simulink model "B2B_2x15kW_LCO_paralelo_y_serie"  (R2026b)
settings: Solver=ode5  StopTime=inf  EnableMultiTasking=on
StopFcn:
  | Modelo_Disable_B2B
undefined symbols (not defined in the file): ALPHA_DC, COS_RO, dataStateMachine, DiscIntNeverNeededParam, dq2abc, EN_G, getNormalizedOffset, I_MAX_G, INV_SIN_RO, KAW_CCG, KAW_DC, KI_CCG, KI_DC, KI_PLLG, KP_CCG, KP_DC, KP_PLLG, L12, LIMIT_SAG_DETECT, magnitude, MIN_VDC_READY, Ncount, NDELAY_SAG_DETECT, PORC_DC_STEADS, SAMPLES_SAG_DETECT, simDCcontCurrent1, simDCcontCurrent2, SN_G, Transformations_blocks, ts, Ts_al, TS_C, TS_PLL, UDC_min_al, UDC_Ref_al, VDC_REF, WN_G
libraries: simulink x15, TriPhaseDriveControl x13, powerlib_extras x2, model_hardware_PM15F80C_rev x2, TriphaseXenomaiTarget x1
(part 1 of 4)
settings Model: ExtModeArchiveDirName=C:\Users\erick.vazquez\Desktop\Modelos serie-paralelo LCOs-FLL  ExtModeArchiveFileName=Inicializacion_paralelo_serie  ExtModeTrigDirection=either  ExtModeTrigElement=1  SimulationMode=external  Creator=francisco.huerta  LastModifiedBy=ERICK
settings DataIOCC: LimitDataPoints=on  ReturnWorkspaceOutputs=off  SaveFormat=Array  SignalLoggingSaveFormat=ModelDataLogs
settings OptimizationCC: BlockReduction=off  BufferReuse=off  ExpressionFolding=off  GlobalBufferReuse=off  LifeSpan=inf  LocalBlockOutputs=off  OptimizeBlockIOStorage=off
settings DebuggingCC: ArithmeticOperatorsInVariantConditions=warning  MergeDetectMultiDrivingBlocksExec=none  MultiTaskCondExecSysMsg=none  MultiTaskDSMMsg=warning  SFExecutionAtInitializationDiag=none  SFNoUnconditionalDefaultTransitionDiag=warning  SFUnexpectedBacktrackingDiag=warning  SolverPrmCheckMsg=warning  StateNameClashWarn=warning  UnderspecifiedInitializationDetection=Classic
settings HardwareCC: ProdEndianess=Unspecified  ProdHWDeviceType=Generic->64-bit Embedded Processor (LP64)  ProdIntDivRoundTo=Undefined  ProdLargestAtomicFloat=None
settings ModelReferenceCC: PropagateSignalLabelsOutOfModel=off
settings SFSimCC: CustomCodeUndefinedFunction=UseInterfaceOnly  SimUseLocalCustomCode=off
settings RTWCC: Description=Linux/Xenomai Native Real-Time Target  RTWUseLocalCustomCode=off  SystemTargetFile=xenomai.tlc  TemplateMakefile=xenomai.tmf
settings CodeAppCC: StateflowObjectComments=on
settings STFCustomTargetCC: CPPClassGenCompliant=on  CodeReplacementLibrary=GNU  ModelReferenceCompliant=off  SystemTargetFile=xenomai.tlc
settings GRTTargetCC: CodeReplacementLibrary=GNU  CombineOutputUpdateFcns=off  CompOptLevelCompliant=off  ConcurrentExecutionCompliant=off  ExtMode=on  ExtModeMexArgs='10.0.14.31', 0, 17725  GRTInterface=on  MatFileLogging=off  ModelReferenceCompliant=off  ParMdlRefBuildCompliant=off
settings ConfigComp: CovExternalEMLEnable=off  CovSFcnEnable=off  CovSaveCumulativeToWorkspaceVar=on  CovSaveSingleToWorkspaceVar=on

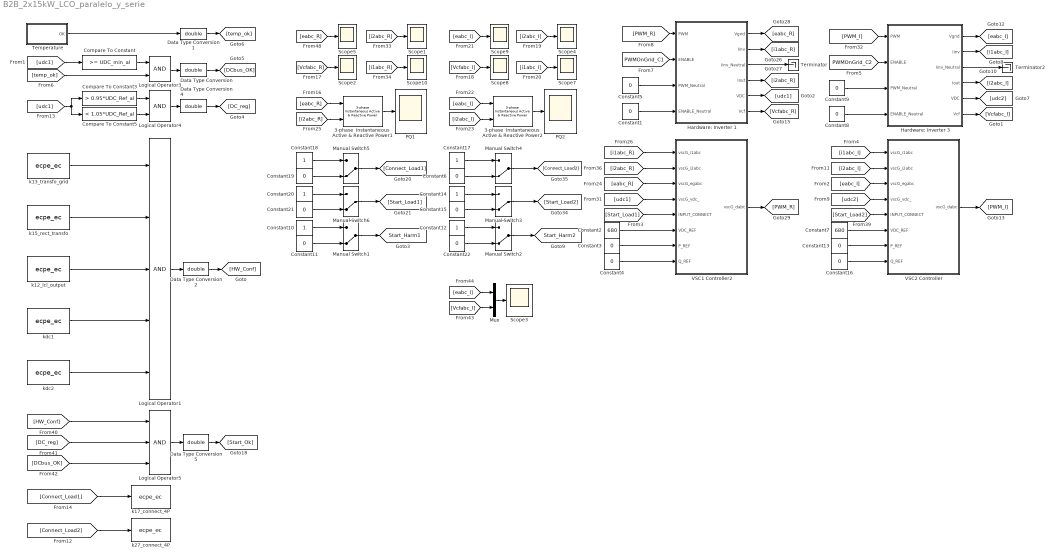
== system B2B_2x15kW_LCO_paralelo_y_serie ==
  3-phase  Instantaneous  Active & Reactive Power1 : powerlib_extras/Measurements/3-phase  Instantaneous  Active & Reactive Power
  3-phase  Instantaneous  Active & Reactive Power2 : powerlib_extras/Measurements/3-phase  Instantaneous  Active & Reactive Power
  Compare To Constant : simulink/Logic and Bit Operations/Compare To Constant  relop=>=  const=UDC_min_al  OutDataTypeStr=boolean
  Compare To Constant3 : simulink/Logic and Bit Operations/Compare To Constant  relop=>  const=0.95*UDC_Ref_al  OutDataTypeStr=boolean
  Compare To Constant5 : simulink/Logic and Bit Operations/Compare To Constant  relop=<  const=1.05*UDC_Ref_al  OutDataTypeStr=boolean
  Constant{1,3..6,8..9,11,13,15..16,19,21..22} (14 alike) : Constant  Value=0
  Constant{10,12,14,17..18,20} (6 alike) : Constant
  Constant2 : Constant  Value=680
  Constant7 : Constant  Value=680
  Data Type Conversion{,1..2,4..5} (5 alike) : DataTypeConversion  OutDataTypeStr=double  SaturateOnIntegerOverflow=off  RndMeth=Floor
  Hardware: Inverter 1 : Subsystem
  Hardware: Inverter 3 : Subsystem
  Logical Operator1 : Logic  Inputs=5  AllPortsSameDT=off  OutDataTypeStr=boolean  SampleTime=Ts_al
  Logical Operator3 : Logic  AllPortsSameDT=off  OutDataTypeStr=boolean  SampleTime=Ts_al
  Logical Operator4 : Logic  AllPortsSameDT=off  OutDataTypeStr=boolean  SampleTime=Ts_al
  Logical Operator5 : Logic  Inputs=3  AllPortsSameDT=off  OutDataTypeStr=boolean  SampleTime=Ts_al
  Manual Switch{1..6} (6 alike) : ManualSwitch  CurrentSetting=0
  Mux : Mux  Inputs=2
  PQ1 : Scope
      settings: TimeSpan=1  ActiveDisplayYMinimum=-200  ActiveDisplayYMaximum=1200  DataLoggingMaxPoints=10000  DataLoggingVariableName=Potencias_C1
  PQ2 : Scope
      settings: TimeSpan=10  ActiveDisplayYMinimum=-1750  ActiveDisplayYMaximum=3000  DataLoggingMaxPoints=10000  DataLoggingVariableName=Potencias_C2
  Scope{1..5,7..10} (9 alike) : Scope
      Scope1 settings: TimeSpan=0.1  ActiveDisplayYMinimum=-6  ActiveDisplayYMaximum=6  DataLoggingVariableName=I2_1_abc
      Scope10 settings: TimeSpan=0.1  DataLoggingVariableName=MedidasTrifasicas1
      Scope2 settings: TimeSpan=0.04  ActiveDisplayYMinimum=-400  ActiveDisplayYMaximum=400  DataLoggingVariableName=MedidasTrifasicas3
      Scope3 settings: TimeSpan=0.04  ActiveDisplayYMinimum=-700  ActiveDisplayYMaximum=800  DataLoggingVariableName=MedidasTrifasicas
      Scope4 settings: TimeSpan=0.04  ActiveDisplayYMinimum=-3.5  ActiveDisplayYMaximum=4  DataLoggingVariableName=I2_2_abc
      Scope5 settings: TimeSpan=0.04  ActiveDisplayYMinimum=-350  ActiveDisplayYMaximum=350  DataLoggingVariableName=Vpcc1_abc
      Scope7 settings: TimeSpan=0.1  ActiveDisplayYMinimum=-0.45  ActiveDisplayYMaximum=0.025  DataLoggingVariableName=MedidasTrifasicas5
      Scope8 settings: TimeSpan=0.1  ActiveDisplayYMinimum=-0.5  ActiveDisplayYMaximum=3.5  DataLoggingVariableName=MedidasTrifasicas6
      Scope9 settings: TimeSpan=0.04  ActiveDisplayYMinimum=-2  ActiveDisplayYMaximum=6  DataLoggingVariableName=Vpcc2_abc
  Temperature : Subsystem
  Terminator : Terminator
  Terminator2 : Terminator
  VSC1 Controller2 : Subsystem
  VSC2 Controller : Subsystem
  k12_lcl_output : TriPhaseDriveControl/Hardware/ecpe_ec  sampletime=Ts_al  names_out='k12_lcl_output'  names_in=''  use_default_values=on  out_values=[]
  k13_transfo_grid : TriPhaseDriveControl/Hardware/ecpe_ec  sampletime=Ts_al  names_out='k13_transfo_grid'  names_in=''  use_default_values=on  out_values=[]
  k15_rect_transfo : TriPhaseDriveControl/Hardware/ecpe_ec  sampletime=Ts_al  names_out='k15_rect_transfo'  names_in=''  use_default_values=on  out_values=[]
  k17_connect_4P : TriPhaseDriveControl/Hardware/ecpe_ec  sampletime=Ts_al  names_out=''  names_in='k17_connect_4P'  use_default_values=on  out_values=[]
  k27_connect_4P : TriPhaseDriveControl/Hardware/ecpe_ec  sampletime=Ts_al  names_out=''  names_in='k27_connect_4P'  use_default_values=on  out_values=[]
  kdc1 : TriPhaseDriveControl/Hardware/ecpe_ec  sampletime=Ts_al  names_out='kdc1'  names_in=''  use_default_values=on  out_values=[]
  kdc2 : TriPhaseDriveControl/Hardware/ecpe_ec  sampletime=Ts_al  names_out='kdc2'  names_in=''  use_default_values=on  out_values=[]
  tag scope: Start_Harm1=global, Start_Harm2=global
  wires:
  Logical Operator1/1 -> Data Type Conversion2/1
  [udc1] -> Compare To Constant/1
  Compare To Constant/1 -> Logical Operator3/1
  Logical Operator3/1 -> Data Type Conversion/1
  [temp_ok] -> Logical Operator3/2
  Temperature/1(OK) -> Data Type Conversion1/1
  Data Type Conversion/1 -> [DCbus_OK]
  Data Type Conversion1/1 -> [temp_ok]
  Data Type Conversion2/1 -> [HW_Conf]
  [udc1] -> Compare To Constant3/1, Compare To Constant5/1
  Compare To Constant3/1 -> Logical Operator4/1
  Compare To Constant5/1 -> Logical Operator4/2
  Data Type Conversion4/1 -> [DC_reg]
  Logical Operator4/1 -> Data Type Conversion4/1
  [Vcfabc_R] -> Scope2/1
  [eabc_R] -> Scope5/1
  Constant5/1 -> Hardware: Inverter 1/3(PWM_Neutral)
  Constant1/1 -> Hardware: Inverter 1/4(ENABLE_Neutral)
  Hardware: Inverter 1/1(Vgrid) -> [eabc_R]
  Hardware: Inverter 1/2(Iinv) -> [i1abc_R]
  Hardware: Inverter 1/3(Iinv_Neutral) -> Terminator/1
  Hardware: Inverter 1/4(Iout) -> [i2abc_R]
  Hardware: Inverter 1/5(VDC) -> [udc1]
  Hardware: Inverter 1/6(Vcf) -> [Vcfabc_R]
  Manual Switch3/1 -> [Start_Load2]
  Manual Switch4/1 -> [Connect_Load2]
  Constant14/1 -> Manual Switch3/1
  Constant15/1 -> Manual Switch3/2
  Constant6/1 -> Manual Switch4/2
  Constant17/1 -> Manual Switch4/1
  [i2abc_R] -> Scope1/1
  Hardware: Inverter 3/1(Vgrid) -> [eabc_I]
  Hardware: Inverter 3/4(Iout) -> [i2abc_I]
  Hardware: Inverter 3/2(Iinv) -> [i1abc_I]
  Hardware: Inverter 3/6(Vcf) -> [Vcfabc_I]
  Hardware: Inverter 3/5(VDC) -> [udc2]
  Hardware: Inverter 3/3(Iinv_Neutral) -> Terminator2/1
  Constant9/1 -> Hardware: Inverter 3/3(PWM_Neutral)
  Constant8/1 -> Hardware: Inverter 3/4(ENABLE_Neutral)
  [eabc_R] -> 3-phase  Instantaneous  Active & Reactive Power1/1
  [i2abc_R] -> 3-phase  Instantaneous  Active & Reactive Power1/2
  3-phase  Instantaneous  Active & Reactive Power1/1 -> PQ1/1
  [i1abc_R] -> Scope10/1
  VSC2 Controller/1(vscG_dabc) -> [PWM_I]
  [i1abc_I] -> VSC2 Controller/1(vscG_i1abc)
  [i2abc_I] -> VSC2 Controller/2(vscG_i2abc)
  [eabc_I] -> VSC2 Controller/3(vscG_egabc)
  [udc2] -> VSC2 Controller/4(vscG_vdc_)
  Constant16/1 -> VSC2 Controller/8(Q_REF)
  Constant13/1 -> VSC2 Controller/7(P_REF)
  [Connect_Load2] -> k27_connect_4P/1
  [Vcfabc_I] -> Scope8/1
  [eabc_I] -> Scope9/1
  [i2abc_I] -> Scope4/1
  [i1abc_I] -> Scope7/1
  [eabc_I] -> 3-phase  Instantaneous  Active & Reactive Power2/1
  [i2abc_I] -> 3-phase  Instantaneous  Active & Reactive Power2/2
  3-phase  Instantaneous  Active & Reactive Power2/1 -> PQ2/1
  [Start_Load2] -> VSC2 Controller/5(INPUT_CONNECT)
  [HW_Conf] -> Logical Operator5/1
  [DC_reg] -> Logical Operator5/2
  [DCbus_OK] -> Logical Operator5/3
  Logical Operator5/1 -> Data Type Conversion5/1
  Data Type Conversion5/1 -> [Start_Ok]
  Manual Switch5/1 -> [Connect_Load1]
  Manual Switch6/1 -> [Start_Load1]
  Constant18/1 -> Manual Switch5/1
  Constant19/1 -> Manual Switch5/2
  Constant21/1 -> Manual Switch6/2
  Constant20/1 -> Manual Switch6/1
  Mux/1 -> Scope3/1
  [eabc_I] -> Mux/1
  [Vcfabc_I] -> Mux/2
  [Connect_Load1] -> k17_connect_4P/1
  VSC1 Controller2/1(vscG_dabc) -> [PWM_R]
  Constant3/1 -> VSC1 Controller2/7(P_REF)
  Constant4/1 -> VSC1 Controller2/8(Q_REF)
  [i2abc_R] -> VSC1 Controller2/2(vscG_i2abc)
  [Start_Load1] -> VSC1 Controller2/5(INPUT_CONNECT)
  [i1abc_R] -> VSC1 Controller2/1(vscG_i1abc)
  [udc1] -> VSC1 Controller2/4(vscG_vdc_)
  [eabc_R] -> VSC1 Controller2/3(vscG_egabc)
  Constant2/1 -> VSC1 Controller2/6(VDC_REF)
  Constant7/1 -> VSC2 Controller/6(VDC_REF)
  k13_transfo_grid/1 -> Logical Operator1/1
  k15_rect_transfo/1 -> Logical Operator1/2
  k12_lcl_output/1 -> Logical Operator1/3
  kdc2/1 -> Logical Operator1/5
  kdc1/1 -> Logical Operator1/4
  [PWMOnGrid_C1] -> Hardware: Inverter 1/2(ENABLE)
  [PWMOnGrid_C2] -> Hardware: Inverter 3/2(ENABLE)
  [PWM_R] -> Hardware: Inverter 1/1(PWM)
  [PWM_I] -> Hardware: Inverter 3/1(PWM)
  Manual Switch1/1 -> [Start_Harm1]
  Constant11/1 -> Manual Switch1/2
  Constant10/1 -> Manual Switch1/1
  Manual Switch2/1 -> [Start_Harm2]
  Constant22/1 -> Manual Switch2/2
  Constant12/1 -> Manual Switch2/1

== system B2B_2x15kW_LCO_paralelo_y_serie/Hardware: Inverter 1 ==
  PWM : Inport
  ENABLE : Inport  Port=2
  PWM_Neutral : Inport  Port=3
  ENABLE_Neutral : Inport  Port=4
  Hardware: 3ph + N (Inverter 1) no termination inv3 : model_hardware_PM15F80C_rev/Hardware: 3ph + N (Inverter 1) no termination inv3  Ts=Ts_al  DT=DT_al  ack=0
  Off-set : Subsystem
  Off-set1 : Subsystem
  Off-set2 : Subsystem
  Off-set3 : Subsystem
  Voltage1 : TriPhaseDriveControl/Hardware/Voltage  Ts=ts  devNames='INVERTER_1/U/M4/CH10,INVERTER_1/U/M4/CH11,INVERTER_1/U/M4/CH12'  vLimOn=off  vLim=600  vFilt=none  vRange=1000  vOffs=getNormalizedOffset([0 0 0], 1000, 1/8000)
  Vgrid : Outport
  Iinv : Outport  Port=2
  Iinv_Neutral : Outport  Port=3
  Iout : Outport  Port=4
  VDC : Outport  Port=5
  Vcf : Outport  Port=6
  wires:
  PWM_Neutral/1 -> Hardware: 3ph + N (Inverter 1) no termination inv3/3
  Hardware: 3ph + N (Inverter 1) no termination inv3/5 -> VDC/1
  ENABLE/1 -> Hardware: 3ph + N (Inverter 1) no termination inv3/2
  PWM/1 -> Hardware: 3ph + N (Inverter 1) no termination inv3/1
  ENABLE_Neutral/1 -> Hardware: 3ph + N (Inverter 1) no termination inv3/4
  Hardware: 3ph + N (Inverter 1) no termination inv3/2 -> Off-set1/1(In)
  Hardware: 3ph + N (Inverter 1) no termination inv3/4 -> Off-set/1(In)
  Hardware: 3ph + N (Inverter 1) no termination inv3/1 -> Off-set2/1(In)
  Voltage1/1 -> Off-set3/1(In)
  Off-set2/1(Out) -> Vgrid/1
  Off-set1/1(Out) -> Iinv/1
  Hardware: 3ph + N (Inverter 1) no termination inv3/3 -> Iinv_Neutral/1
  Off-set/1(Out) -> Iout/1
  Off-set3/1(Out) -> Vcf/1

== system B2B_2x15kW_LCO_paralelo_y_serie/Hardware: Inverter 3 ==
  PWM : Inport
  ENABLE : Inport  Port=2
  PWM_Neutral : Inport  Port=3
  ENABLE_Neutral : Inport  Port=4
  Hardware: 3ph + N (Inverter 3) no termination inv1 : model_hardware_PM15F80C_rev/Hardware: 3ph + N (Inverter 3) no termination inv1  Ts=Ts_al  DT=DT_al  ack=0
  Off-set : Subsystem
  Off-set1 : Subsystem
  Off-set2 : Subsystem
  Off-set3 : Subsystem
  Voltage1 : TriPhaseDriveControl/Hardware/Voltage  Ts=ts  devNames='INVERTER_3/U/M4/CH10,INVERTER_3/U/M4/CH11,INVERTER_3/U/M4/CH12'  vLimOn=off  vLim=600  vFilt=none  vRange=1000  vOffs=getNormalizedOffset([0 0 0], 1000, 1/8000)
  Vgrid : Outport
  Iinv : Outport  Port=2
  Iinv_Neutral : Outport  Port=3
  Iout : Outport  Port=4
  VDC : Outport  Port=5
  Vcf : Outport  Port=6
  wires:
  Voltage1/1 -> Off-set3/1(In)
  Hardware: 3ph + N (Inverter 3) no termination inv1/1 -> Off-set2/1(In)
  Hardware: 3ph + N (Inverter 3) no termination inv1/3 -> Iinv_Neutral/1
  Hardware: 3ph + N (Inverter 3) no termination inv1/4 -> Off-set/1(In)
  Hardware: 3ph + N (Inverter 3) no termination inv1/2 -> Off-set1/1(In)
  ENABLE_Neutral/1 -> Hardware: 3ph + N (Inverter 3) no termination inv1/4
  PWM/1 -> Hardware: 3ph + N (Inverter 3) no termination inv1/1
  ENABLE/1 -> Hardware: 3ph + N (Inverter 3) no termination inv1/2
  Hardware: 3ph + N (Inverter 3) no termination inv1/5 -> VDC/1
  PWM_Neutral/1 -> Hardware: 3ph + N (Inverter 3) no termination inv1/3
  Off-set1/1(Out) -> Iinv/1
  Off-set/1(Out) -> Iout/1
  Off-set2/1(Out) -> Vgrid/1
  Off-set3/1(Out) -> Vcf/1

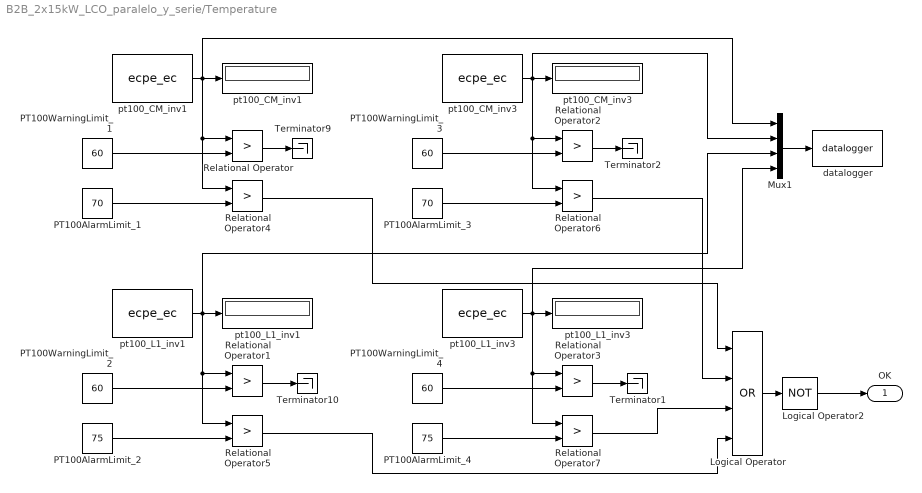
== system B2B_2x15kW_LCO_paralelo_y_serie/Temperature ==
  Logical Operator : Logic  Operator=OR  Inputs=4  AllPortsSameDT=off  OutDataTypeStr=boolean
  Logical Operator2 : Logic  Operator=NOT  AllPortsSameDT=off  OutDataTypeStr=boolean
  Mux1 : Mux
  PT100AlarmLimit_1 : Constant  Value=70
  PT100AlarmLimit_2 : Constant  Value=75
  PT100AlarmLimit_3 : Constant  Value=70
  PT100AlarmLimit_4 : Constant  Value=75
  PT100WarningLimit_{1..4} (4 alike) : Constant  Value=60
  Relational Operator{,1..7} (8 alike) : RelationalOperator  Operator=>  OutDataTypeStr=boolean  InputSameDT=off
  Terminator{1..2,9..10} (4 alike) : Terminator
  datalogger : TriphaseXenomaiTarget/datalogger  memoryName=triphase_temperature  decimation=1/Ts_al*0.5  sampleTime=Ts_al
  pt100_CM_inv1 : TriPhaseDriveControl/Hardware/ecpe_ec  sampletime=Ts_al  names_out='pt100_CM_inv1'  names_in=''  use_default_values=on  out_values=[]
  "pt100_CM_inv1 " : Display
      settings: Decimation=round(0.5/ts)
  pt100_CM_inv3 : TriPhaseDriveControl/Hardware/ecpe_ec  sampletime=Ts_al  names_out='pt100_CM_inv3'  names_in=''  use_default_values=on  out_values=[]
  "pt100_CM_inv3 " : Display
      settings: Decimation=round(0.5/ts)
  pt100_L1_inv1 : TriPhaseDriveControl/Hardware/ecpe_ec  sampletime=Ts_al  names_out='pt100_L1_inv1'  names_in=''  use_default_values=on  out_values=[]
  "pt100_L1_inv1 " : Display
      settings: Decimation=round(0.5/ts)
  pt100_L1_inv3 : TriPhaseDriveControl/Hardware/ecpe_ec  sampletime=Ts_al  names_out='pt100_L1_inv3'  names_in=''  use_default_values=on  out_values=[]
  "pt100_L1_inv3 " : Display
      settings: Decimation=round(0.5/ts)
  OK : Outport
  wires:
  pt100_CM_inv1/1 -> "pt100_CM_inv1 "/1, Relational Operator/1, Relational Operator4/1, Mux1/1
  pt100_L1_inv1/1 -> "pt100_L1_inv1 "/1, Relational Operator1/1, Relational Operator5/1, Mux1/3
  PT100WarningLimit_1/1 -> Relational Operator/2
  Relational Operator/1 -> Terminator9/1
  PT100WarningLimit_2/1 -> Relational Operator1/2
  Relational Operator1/1 -> Terminator10/1
  PT100AlarmLimit_1/1 -> Relational Operator4/2
  PT100AlarmLimit_2/1 -> Relational Operator5/2
  Logical Operator/1 -> Logical Operator2/1
  Logical Operator2/1 -> OK/1
  pt100_CM_inv3/1 -> "pt100_CM_inv3 "/1, Relational Operator2/1, Relational Operator6/1, Mux1/2
  pt100_L1_inv3/1 -> "pt100_L1_inv3 "/1, Relational Operator3/1, Relational Operator7/1, Mux1/4
  PT100WarningLimit_3/1 -> Relational Operator2/2
  Relational Operator2/1 -> Terminator2/1
  PT100WarningLimit_4/1 -> Relational Operator3/2
  Relational Operator3/1 -> Terminator1/1
  PT100AlarmLimit_3/1 -> Relational Operator6/2
  PT100AlarmLimit_4/1 -> Relational Operator7/2
  Relational Operator4/1 -> Logical Operator/1
  Relational Operator6/1 -> Logical Operator/2
  Relational Operator5/1 -> Logical Operator/4
  Relational Operator7/1 -> Logical Operator/3
  Mux1/1 -> datalogger/1

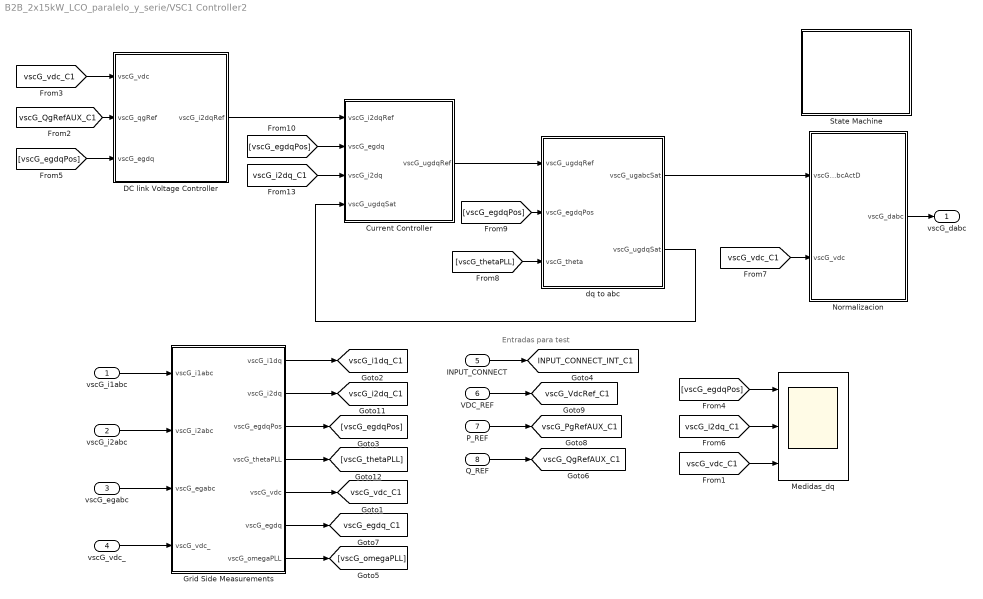
== system B2B_2x15kW_LCO_paralelo_y_serie/VSC1 Controller2 ==
  note: Entradas para test
  vscG_i1abc : Inport  SampleTime=TS_C
  vscG_i2abc : Inport  Port=2  SampleTime=TS_C
  vscG_egabc : Inport  Port=3  SampleTime=TS_PLL
  vscG_vdc_ : Inport  Port=4  SampleTime=TS_C
  INPUT_CONNECT : Inport  Port=5  SampleTime=TS_PLL
  VDC_REF : Inport  Port=6  SampleTime=TS_PLL
  P_REF : Inport  Port=7  SampleTime=TS_PLL
  Q_REF : Inport  Port=8  SampleTime=TS_PLL
  Current Controller : Subsystem
  DC link Voltage Controller : Subsystem
  Grid Side Measurements : Subsystem
  Medidas_dq : Scope  NumInputPorts=3
      settings: TimeSpan=5  ActiveDisplayYMinimum=-200  ActiveDisplayYMaximum=225  DataLoggingVariableName=MedidasDQ_C1
  Normalizacion : Subsystem
  State Machine : Subsystem
  dq to abc : Subsystem
  vscG_dabc : Outport
  tag scope: INPUT_CONNECT_INT_C1=global, vscG_PgRefAUX_C1=global, vscG_QgRefAUX_C1=global, vscG_VdcRef_C1=global, vscG_egdq_C1=global, vscG_i1dq_C1=global, vscG_i2dq_C1=global, vscG_vdc_C1=global
  wires:
  vscG_i1abc/1 -> Grid Side Measurements/1(vscG_i1abc)
  vscG_i2abc/1 -> Grid Side Measurements/2(vscG_i2abc)
  vscG_egabc/1 -> Grid Side Measurements/3(vscG_egabc)
  Grid Side Measurements/3(vscG_egdqPos) -> [vscG_egdqPos]
  DC link Voltage Controller/1(vscG_i2dqRef) -> Current Controller/1(vscG_i2dqRef)
  Current Controller/1(vscG_ugdqRef) -> dq to abc/1(vscG_ugdqRef)
  [vscG_egdqPos] -> DC link Voltage Controller/3(vscG_egdq)
  vscG_vdc_/1 -> Grid Side Measurements/4(vscG_vdc_)
  [vscG_vdc_C1] -> DC link Voltage Controller/1(vscG_vdc)
  Grid Side Measurements/6(vscG_egdq) -> [vscG_egdq_C1]
  Grid Side Measurements/7(vscG_omegaPLL) -> [vscG_omegaPLL]
  Grid Side Measurements/5(vscG_vdc) -> [vscG_vdc_C1]
  [vscG_vdc_C1] -> Normalizacion/2(vscG_vdc)
  Normalizacion/1(vscG_dabc) -> vscG_dabc/1
  INPUT_CONNECT/1 -> [INPUT_CONNECT_INT_C1]
  VDC_REF/1 -> [vscG_VdcRef_C1]
  P_REF/1 -> [vscG_PgRefAUX_C1]
  Q_REF/1 -> [vscG_QgRefAUX_C1]
  Grid Side Measurements/1(vscG_i1dq) -> [vscG_i1dq_C1]
  Grid Side Measurements/4(vscG_thetaPLL) -> [vscG_thetaPLL]
  Grid Side Measurements/2(vscG_i2dq) -> [vscG_i2dq_C1]
  [vscG_egdqPos] -> Current Controller/2(vscG_egdq)
  [vscG_i2dq_C1] -> Current Controller/3(vscG_i2dq)
  [vscG_thetaPLL] -> dq to abc/3(vscG_theta)
  [vscG_QgRefAUX_C1] -> DC link Voltage Controller/2(vscG_qgRef)
  [vscG_vdc_C1] -> Medidas_dq/3
  [vscG_i2dq_C1] -> Medidas_dq/2
  [vscG_egdqPos] -> Medidas_dq/1
  dq to abc/1(vscG_ugabcSat) -> Normalizacion/1(vscG_ugabcActD)
  [vscG_egdqPos] -> dq to abc/2(vscG_egdqPos)
  dq to abc/2(vscG_ugdqSat) -> Current Controller/4(vscG_ugdqSat)

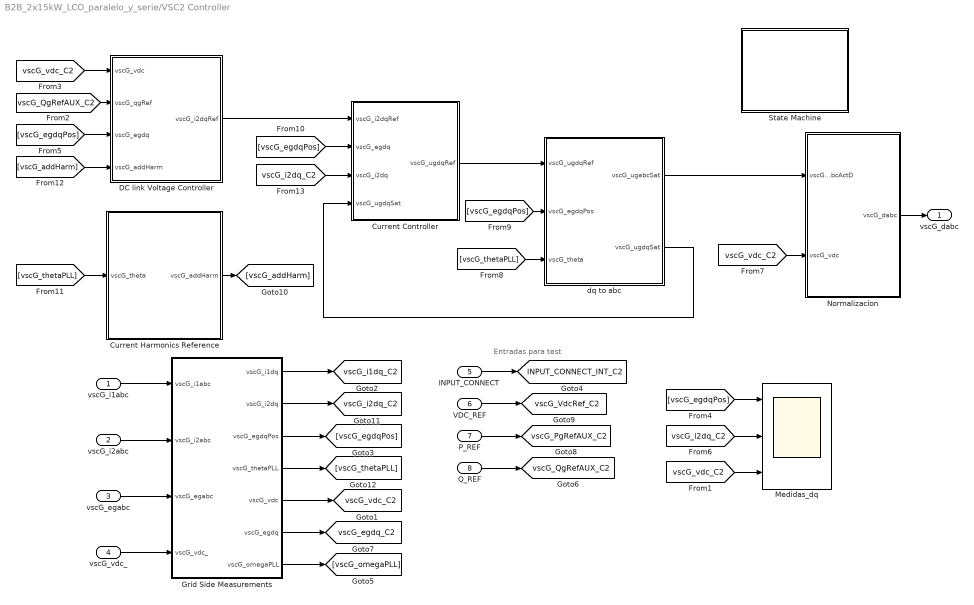
== system B2B_2x15kW_LCO_paralelo_y_serie/VSC2 Controller ==
  note: Entradas para test
  vscG_i1abc : Inport  SampleTime=TS_C
  vscG_i2abc : Inport  Port=2  SampleTime=TS_C
  vscG_egabc : Inport  Port=3  SampleTime=TS_PLL
  vscG_vdc_ : Inport  Port=4  SampleTime=TS_C
  INPUT_CONNECT : Inport  Port=5  SampleTime=TS_PLL
  VDC_REF : Inport  Port=6  SampleTime=TS_PLL
  P_REF : Inport  Port=7  SampleTime=TS_PLL
  Q_REF : Inport  Port=8  SampleTime=TS_PLL
  Current Controller : Subsystem
  Current Harmonics Reference : Subsystem
  DC link Voltage Controller : Subsystem
  Grid Side Measurements : Subsystem
  Medidas_dq : Scope  NumInputPorts=3
      settings: TimeSpan=10  ActiveDisplayYMinimum=320  ActiveDisplayYMaximum=350  DataLoggingVariableName=MedidasDQ_C2
  Normalizacion : Subsystem
  State Machine : Subsystem
  dq to abc : Subsystem
  vscG_dabc : Outport
  tag scope: INPUT_CONNECT_INT_C2=global, vscG_PgRefAUX_C2=global, vscG_QgRefAUX_C2=global, vscG_VdcRef_C2=global, vscG_egdq_C2=global, vscG_i1dq_C2=global, vscG_i2dq_C2=global, vscG_vdc_C2=global
  wires:
  vscG_i1abc/1 -> Grid Side Measurements/1(vscG_i1abc)
  vscG_i2abc/1 -> Grid Side Measurements/2(vscG_i2abc)
  vscG_egabc/1 -> Grid Side Measurements/3(vscG_egabc)
  Grid Side Measurements/3(vscG_egdqPos) -> [vscG_egdqPos]
  DC link Voltage Controller/1(vscG_i2dqRef) -> Current Controller/1(vscG_i2dqRef)
  Current Controller/1(vscG_ugdqRef) -> dq to abc/1(vscG_ugdqRef)
  [vscG_egdqPos] -> DC link Voltage Controller/3(vscG_egdq)
  vscG_vdc_/1 -> Grid Side Measurements/4(vscG_vdc_)
  [vscG_vdc_C2] -> DC link Voltage Controller/1(vscG_vdc)
  Grid Side Measurements/6(vscG_egdq) -> [vscG_egdq_C2]
  Grid Side Measurements/7(vscG_omegaPLL) -> [vscG_omegaPLL]
  Grid Side Measurements/5(vscG_vdc) -> [vscG_vdc_C2]
  [vscG_vdc_C2] -> Normalizacion/2(vscG_vdc)
  Normalizacion/1(vscG_dabc) -> vscG_dabc/1
  INPUT_CONNECT/1 -> [INPUT_CONNECT_INT_C2]
  VDC_REF/1 -> [vscG_VdcRef_C2]
  P_REF/1 -> [vscG_PgRefAUX_C2]
  Q_REF/1 -> [vscG_QgRefAUX_C2]
  Grid Side Measurements/1(vscG_i1dq) -> [vscG_i1dq_C2]
  Grid Side Measurements/4(vscG_thetaPLL) -> [vscG_thetaPLL]
  Grid Side Measurements/2(vscG_i2dq) -> [vscG_i2dq_C2]
  [vscG_egdqPos] -> Current Controller/2(vscG_egdq)
  [vscG_i2dq_C2] -> Current Controller/3(vscG_i2dq)
  [vscG_thetaPLL] -> dq to abc/3(vscG_theta)
  [vscG_QgRefAUX_C2] -> DC link Voltage Controller/2(vscG_qgRef)
  [vscG_vdc_C2] -> Medidas_dq/3
  [vscG_i2dq_C2] -> Medidas_dq/2
  [vscG_egdqPos] -> Medidas_dq/1
  dq to abc/1(vscG_ugabcSat) -> Normalizacion/1(vscG_ugabcActD)
  [vscG_egdqPos] -> dq to abc/2(vscG_egdqPos)
  dq to abc/2(vscG_ugdqSat) -> Current Controller/4(vscG_ugdqSat)
  Current Harmonics Reference/1(vscG_addHarm) -> [vscG_addHarm]
  [vscG_thetaPLL] -> Current Harmonics Reference/1(vscG_theta)
  [vscG_addHarm] -> DC link Voltage Controller/4(vscG_addHarm)

== system B2B_2x15kW_LCO_paralelo_y_serie/Hardware: Inverter 1/Off-set ==
  In : Inport
  Demux1 : Demux  Outputs=3
  Mux1 : Mux  Inputs=3
  Sum : Sum  Inputs=|++
  Sum1 : Sum  Inputs=|++
  Sum2 : Sum  Inputs=|++
  a : Constant  Value=0
  b : Constant  Value=0
  c : Constant  Value=0
  Out : Outport
  wires:
  Mux1/1 -> Out/1
  Demux1/2 -> Sum1/1
  Demux1/1 -> Sum/1
  Sum1/1 -> Mux1/2
  In/1 -> Demux1/1
  Sum/1 -> Mux1/1
  Sum2/1 -> Mux1/3
  Demux1/3 -> Sum2/1
  a/1 -> Sum/2
  b/1 -> Sum1/2
  c/1 -> Sum2/2

== system B2B_2x15kW_LCO_paralelo_y_serie/Hardware: Inverter 1/Off-set1 ==
  In : Inport
  Demux1 : Demux  Outputs=3
  Mux1 : Mux  Inputs=3
  Sum : Sum  Inputs=|++
  Sum1 : Sum  Inputs=|++
  Sum2 : Sum  Inputs=|++
  a : Constant  Value=0
  b : Constant  Value=-0.6
  c : Constant  Value=0.5
  Out : Outport
  wires:
  Mux1/1 -> Out/1
  Demux1/2 -> Sum1/1
  Demux1/1 -> Sum/1
  Sum1/1 -> Mux1/2
  In/1 -> Demux1/1
  Sum/1 -> Mux1/1
  Sum2/1 -> Mux1/3
  Demux1/3 -> Sum2/1
  a/1 -> Sum/2
  b/1 -> Sum1/2
  c/1 -> Sum2/2

== system B2B_2x15kW_LCO_paralelo_y_serie/Hardware: Inverter 1/Off-set2 ==
  In : Inport
  Demux1 : Demux  Outputs=3
  Mux1 : Mux  Inputs=3
  Sum : Sum  Inputs=|++
  Sum1 : Sum  Inputs=|++
  Sum2 : Sum  Inputs=|++
  a : Constant  Value=-3
  b : Constant  Value=-1.5
  c : Constant  Value=0
  Out : Outport
  wires:
  Mux1/1 -> Out/1
  Demux1/2 -> Sum1/1
  Demux1/1 -> Sum/1
  Sum1/1 -> Mux1/2
  In/1 -> Demux1/1
  Sum/1 -> Mux1/1
  Sum2/1 -> Mux1/3
  Demux1/3 -> Sum2/1
  a/1 -> Sum/2
  b/1 -> Sum1/2
  c/1 -> Sum2/2

== system B2B_2x15kW_LCO_paralelo_y_serie/Hardware: Inverter 1/Off-set3 ==
  In : Inport
  Demux1 : Demux  Outputs=3
  Mux1 : Mux  Inputs=3
  Sum : Sum  Inputs=|++
  Sum1 : Sum  Inputs=|++
  Sum2 : Sum  Inputs=|++
  a : Constant  Value=0
  b : Constant  Value=0
  c : Constant  Value=0
  Out : Outport
  wires:
  Mux1/1 -> Out/1
  Demux1/2 -> Sum1/1
  Demux1/1 -> Sum/1
  Sum1/1 -> Mux1/2
  In/1 -> Demux1/1
  Sum/1 -> Mux1/1
  Sum2/1 -> Mux1/3
  Demux1/3 -> Sum2/1
  a/1 -> Sum/2
  b/1 -> Sum1/2
  c/1 -> Sum2/2

== system B2B_2x15kW_LCO_paralelo_y_serie/Hardware: Inverter 3/Off-set ==
  In : Inport
  Demux1 : Demux  Outputs=3
  Mux1 : Mux  Inputs=3
  Sum : Sum  Inputs=|++
  Sum1 : Sum  Inputs=|++
  Sum2 : Sum  Inputs=|++
  a : Constant  Value=0.05
  b : Constant  Value=0.15
  c : Constant  Value=-0.05
  Out : Outport
  wires:
  Mux1/1 -> Out/1
  Demux1/2 -> Sum1/1
  Demux1/1 -> Sum/1
  Sum1/1 -> Mux1/2
  In/1 -> Demux1/1
  Sum/1 -> Mux1/1
  Sum2/1 -> Mux1/3
  Demux1/3 -> Sum2/1
  a/1 -> Sum/2
  b/1 -> Sum1/2
  c/1 -> Sum2/2

== system B2B_2x15kW_LCO_paralelo_y_serie/Hardware: Inverter 3/Off-set1 ==
  In : Inport
  Demux1 : Demux  Outputs=3
  Mux1 : Mux  Inputs=3
  Sum : Sum  Inputs=|++
  Sum1 : Sum  Inputs=|++
  Sum2 : Sum  Inputs=|++
  a : Constant  Value=0.35
  b : Constant  Value=0.05
  c : Constant  Value=0.1
  Out : Outport
  wires:
  Mux1/1 -> Out/1
  Demux1/2 -> Sum1/1
  Demux1/1 -> Sum/1
  Sum1/1 -> Mux1/2
  In/1 -> Demux1/1
  Sum/1 -> Mux1/1
  Sum2/1 -> Mux1/3
  Demux1/3 -> Sum2/1
  a/1 -> Sum/2
  b/1 -> Sum1/2
  c/1 -> Sum2/2

== system B2B_2x15kW_LCO_paralelo_y_serie/Hardware: Inverter 3/Off-set2 ==
  In : Inport
  Demux1 : Demux  Outputs=3
  Mux1 : Mux  Inputs=3
  Sum : Sum  Inputs=|++
  Sum1 : Sum  Inputs=|++
  Sum2 : Sum  Inputs=|++
  a : Constant  Value=3
  b : Constant  Value=0
  c : Constant  Value=2
  Out : Outport
  wires:
  Mux1/1 -> Out/1
  Demux1/2 -> Sum1/1
  Demux1/1 -> Sum/1
  Sum1/1 -> Mux1/2
  In/1 -> Demux1/1
  Sum/1 -> Mux1/1
  Sum2/1 -> Mux1/3
  Demux1/3 -> Sum2/1
  a/1 -> Sum/2
  b/1 -> Sum1/2
  c/1 -> Sum2/2

== system B2B_2x15kW_LCO_paralelo_y_serie/Hardware: Inverter 3/Off-set3 ==
  In : Inport
  Demux1 : Demux  Outputs=3
  Mux1 : Mux  Inputs=3
  Sum : Sum  Inputs=|++
  Sum1 : Sum  Inputs=|++
  Sum2 : Sum  Inputs=|++
  a : Constant
  b : Constant  Value=3.7
  c : Constant  Value=6
  Out : Outport
  wires:
  Mux1/1 -> Out/1
  Demux1/2 -> Sum1/1
  Demux1/1 -> Sum/1
  Sum1/1 -> Mux1/2
  In/1 -> Demux1/1
  Sum/1 -> Mux1/1
  Sum2/1 -> Mux1/3
  Demux1/3 -> Sum2/1
  a/1 -> Sum/2
  b/1 -> Sum1/2
  c/1 -> Sum2/2

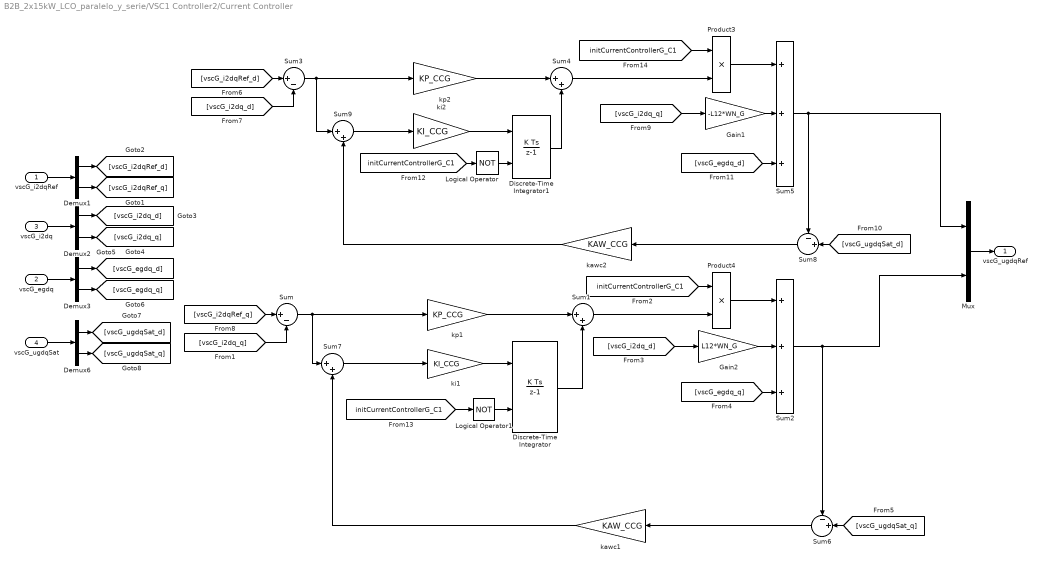
== system B2B_2x15kW_LCO_paralelo_y_serie/VSC1 Controller2/Current Controller ==
  vscG_i2dqRef : Inport
  vscG_egdq : Inport  Port=2
  vscG_i2dq : Inport  Port=3
  vscG_ugdqSat : Inport  Port=4
  Demux{1..3,6} (4 alike) : Demux  Outputs=2
  Discrete-Time Integrator : DiscreteIntegrator  ExternalReset=level  SampleTime=-1  UpperSaturationLimit=sqrt(2/3)*750  LowerSaturationLimit=-sqrt(2/3)*750  ICPrevOutput=DiscIntNeverNeededParam  ICPrevScaledInput=DiscIntNeverNeededParam
  Discrete-Time Integrator1 : DiscreteIntegrator  ExternalReset=level  SampleTime=-1  UpperSaturationLimit=sqrt(2/3)*750  LowerSaturationLimit=-sqrt(2/3)*750  ICPrevOutput=DiscIntNeverNeededParam  ICPrevScaledInput=DiscIntNeverNeededParam
  Gain1 : Gain  Gain=-L12*WN_G  SaturateOnIntegerOverflow=on  OutDataTypeStr=Inherit: Same as input  ParamDataTypeStr=Inherit: Same as input
  Gain2 : Gain  Gain=L12*WN_G  SaturateOnIntegerOverflow=on  OutDataTypeStr=Inherit: Same as input  ParamDataTypeStr=Inherit: Same as input
  Logical Operator : Logic  Operator=NOT  AllPortsSameDT=off  OutDataTypeStr=boolean
  Logical Operator1 : Logic  Operator=NOT  AllPortsSameDT=off  OutDataTypeStr=boolean
  Mux : Mux  Inputs=2
  Product3 : Product  InputSameDT=on  SaturateOnIntegerOverflow=on  OutDataTypeStr=Inherit: Same as first input
  Product4 : Product  InputSameDT=on  SaturateOnIntegerOverflow=on  OutDataTypeStr=Inherit: Same as first input
  Sum : Sum  Inputs=|+-  InputSameDT=on  SaturateOnIntegerOverflow=on  OutDataTypeStr=Inherit: Same as first input
  Sum{1,4,7,9} (4 alike) : Sum  Inputs=|++  InputSameDT=on  SaturateOnIntegerOverflow=on  OutDataTypeStr=Inherit: Same as first input
  Sum2 : Sum  Inputs=+++  InputSameDT=on  SaturateOnIntegerOverflow=on  OutDataTypeStr=Inherit: Same as first input
  Sum3 : Sum  Inputs=|+-  InputSameDT=on  SaturateOnIntegerOverflow=on  OutDataTypeStr=Inherit: Same as first input
  Sum5 : Sum  Inputs=+++  InputSameDT=on  SaturateOnIntegerOverflow=on  OutDataTypeStr=Inherit: Same as first input
  Sum6 : Sum  Inputs=-+|  InputSameDT=on  SaturateOnIntegerOverflow=on  OutDataTypeStr=Inherit: Same as first input
  Sum8 : Sum  Inputs=-+|  InputSameDT=on  SaturateOnIntegerOverflow=on  OutDataTypeStr=Inherit: Same as first input
  kawc1 : Gain  Gain=KAW_CCG  SaturateOnIntegerOverflow=on  OutDataTypeStr=Inherit: Same as input  ParamDataTypeStr=Inherit: Same as input
  kawc2 : Gain  Gain=KAW_CCG  SaturateOnIntegerOverflow=on  OutDataTypeStr=Inherit: Same as input  ParamDataTypeStr=Inherit: Same as input
  ki1 : Gain  Gain=KI_CCG  SaturateOnIntegerOverflow=on  OutDataTypeStr=Inherit: Same as input  ParamDataTypeStr=Inherit: Same as input
  ki2 : Gain  Gain=KI_CCG  SaturateOnIntegerOverflow=on  OutDataTypeStr=Inherit: Same as input  ParamDataTypeStr=Inherit: Same as input
  kp1 : Gain  Gain=KP_CCG  SaturateOnIntegerOverflow=on  OutDataTypeStr=Inherit: Same as input  ParamDataTypeStr=Inherit: Same as input
  kp2 : Gain  Gain=KP_CCG  SaturateOnIntegerOverflow=on  OutDataTypeStr=Inherit: Same as input  ParamDataTypeStr=Inherit: Same as input
  vscG_ugdqRef : Outport
  wires:
  Mux/1 -> vscG_ugdqRef/1
  vscG_i2dq/1 -> Demux2/1
  vscG_egdq/1 -> Demux3/1
  Demux1/1 -> [vscG_i2dqRef_d]
  Demux1/2 -> [vscG_i2dqRef_q]
  Demux2/1 -> [vscG_i2dq_d]
  Demux3/2 -> [vscG_egdq_q]
  Demux3/1 -> [vscG_egdq_d]
  Demux2/2 -> [vscG_i2dq_q]
  vscG_i2dqRef/1 -> Demux1/1
  [vscG_i2dqRef_q] -> Sum/1
  ki1/1 -> Discrete-Time Integrator/1
  [vscG_egdq_q] -> Sum2/3
  Gain2/1 -> Sum2/2
  Sum/1 -> Sum7/1, kp1/1
  [vscG_i2dqRef_d] -> Sum3/1
  ki2/1 -> Discrete-Time Integrator1/1
  Gain1/1 -> Sum5/2
  [vscG_egdq_d] -> Sum5/3
  [vscG_i2dq_q] -> Gain1/1
  Sum3/1 -> Sum9/1, kp2/1
  Logical Operator/1 -> Discrete-Time Integrator1/2
  [initCurrentControllerG_C1] -> Logical Operator/1
  [initCurrentControllerG_C1] -> Logical Operator1/1
  Logical Operator1/1 -> Discrete-Time Integrator/2
  Sum4/1 -> Product3/2
  Product3/1 -> Sum5/1
  [initCurrentControllerG_C1] -> Product3/1
  Product4/1 -> Sum2/1
  Sum1/1 -> Product4/2
  [initCurrentControllerG_C1] -> Product4/1
  [vscG_i2dq_d] -> Sum3/2
  [vscG_i2dq_q] -> Sum/2
  [vscG_i2dq_d] -> Gain2/1
  kp1/1 -> Sum1/1
  Discrete-Time Integrator/1 -> Sum1/2
  Discrete-Time Integrator1/1 -> Sum4/2
  kp2/1 -> Sum4/1
  Sum5/1 -> Sum8/1, Mux/1
  [vscG_ugdqSat_d] -> Sum8/2
  Sum8/1 -> kawc2/1
  Sum9/1 -> ki2/1
  kawc2/1 -> Sum9/2
  Sum2/1 -> Sum6/1, Mux/2
  [vscG_ugdqSat_q] -> Sum6/2
  Sum6/1 -> kawc1/1
  kawc1/1 -> Sum7/2
  Sum7/1 -> ki1/1
  vscG_ugdqSat/1 -> Demux6/1
  Demux6/1 -> [vscG_ugdqSat_d]
  Demux6/2 -> [vscG_ugdqSat_q]

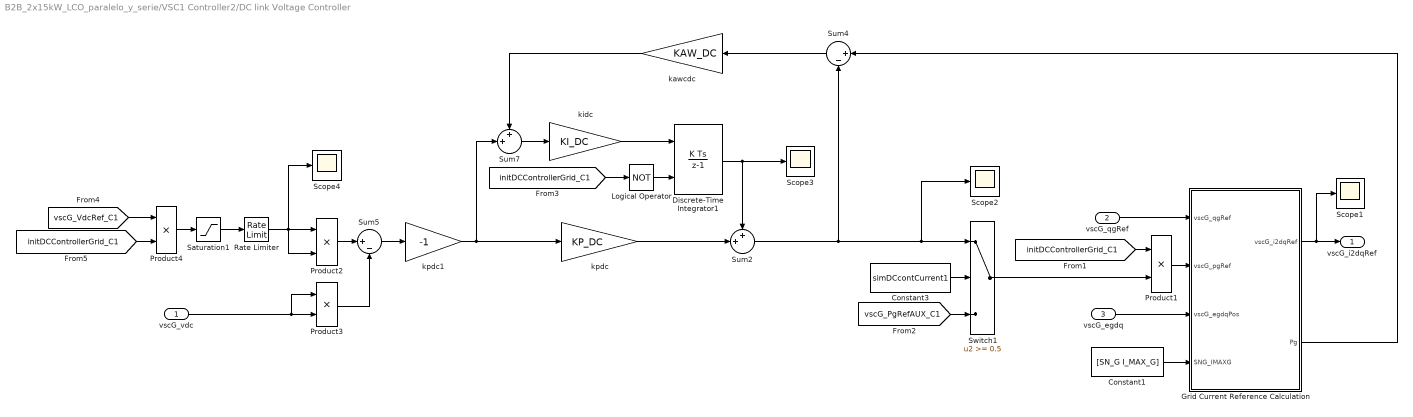
== system B2B_2x15kW_LCO_paralelo_y_serie/VSC1 Controller2/DC link Voltage Controller ==
  vscG_vdc : Inport
  vscG_qgRef : Inport  Port=2
  vscG_egdq : Inport  Port=3
  Constant1 : Constant  Value=[SN_G I_MAX_G]  SampleTime=TS_C
  Constant3 : Constant  Value=simDCcontCurrent1  SampleTime=TS_C
  Discrete-Time Integrator1 : DiscreteIntegrator  ExternalReset=level  SampleTime=-1  UpperSaturationLimit=sqrt(2/3)*750  LowerSaturationLimit=-sqrt(2/3)*750  ICPrevOutput=DiscIntNeverNeededParam  ICPrevScaledInput=DiscIntNeverNeededParam
  Grid Current Reference Calculation : MATLAB Function  TreatAsAtomicUnit=on
  Logical Operator : Logic  Operator=NOT  AllPortsSameDT=off  OutDataTypeStr=boolean
  Product1 : Product  RndMeth=Zero
  Product2 : Product  SaturateOnIntegerOverflow=on  OutDataTypeStr=Inherit: Same as first input
  Product3 : Product  SaturateOnIntegerOverflow=on  OutDataTypeStr=Inherit: Same as first input
  Product4 : Product  SaturateOnIntegerOverflow=on  OutDataTypeStr=Inherit: Same as first input
  Rate Limiter : RateLimiter  RisingSlewLimit=500/1  FallingSlewLimit=-500/1  SampleTimeMode=inherited  InitialCondition=EN_G*sqrt(2)
  Saturation1 : Saturate  UpperLimit=VDC_REF*1.1  LowerLimit=EN_G*sqrt(2)
  Scope{1..4} (4 alike) : Scope
      Scope1 settings: SampleTime=TS_C  TimeSpan=10  ActiveDisplayYMinimum=-0  ActiveDisplayYMaximum=22  DataLoggingDecimation=5  DataLoggingVariableName=Variables_i2dq2  DataLoggingSaveFormat=Array
      Scope2 settings: SampleTime=TS_C  TimeSpan=5  ActiveDisplayYMinimum=-30000  ActiveDisplayYMaximum=2500  DataLoggingDecimation=5  DataLoggingVariableName=Variables_i2dq4  DataLoggingSaveFormat=Array
      Scope3 settings: SampleTime=TS_C  TimeSpan=5  ActiveDisplayYMinimum=24681.8  ActiveDisplayYMaximum=27279.8  DataLoggingDecimation=5  DataLoggingVariableName=Variables_i2dq5  DataLoggingSaveFormat=Array
      Scope4 settings: SampleTime=TS_C  TimeSpan=5  ActiveDisplayYMinimum=675  ActiveDisplayYMaximum=680  DataLoggingDecimation=5  DataLoggingVariableName=Variables_i2dq6  DataLoggingSaveFormat=Array
  Sum2 : Sum  Inputs=++|  InputSameDT=on  SaturateOnIntegerOverflow=on  OutDataTypeStr=Inherit: Same as first input
  Sum4 : Sum  Inputs=|+-  InputSameDT=on  SaturateOnIntegerOverflow=on  OutDataTypeStr=Inherit: Same as first input
  Sum5 : Sum  Inputs=|+-  InputSameDT=on  SaturateOnIntegerOverflow=on  OutDataTypeStr=Inherit: Same as first input
  Sum7 : Sum  Inputs=++|  InputSameDT=on  SaturateOnIntegerOverflow=on  OutDataTypeStr=Inherit: Same as first input
  Switch1 : Switch  Threshold=0.5  SaturateOnIntegerOverflow=off  InputSameDT=off
  kawcdc : Gain  Gain=KAW_DC  SaturateOnIntegerOverflow=on  OutDataTypeStr=Inherit: Same as input  ParamDataTypeStr=Inherit: Same as input
  kidc : Gain  Gain=KI_DC  SaturateOnIntegerOverflow=on  OutDataTypeStr=Inherit: Same as input  ParamDataTypeStr=Inherit: Same as input
  kpdc : Gain  Gain=KP_DC  SaturateOnIntegerOverflow=on  OutDataTypeStr=Inherit: Same as input  ParamDataTypeStr=Inherit: Same as input
  kpdc1 : Gain  Gain=-1  SaturateOnIntegerOverflow=on  OutDataTypeStr=Inherit: Same as input  ParamDataTypeStr=Inherit: Same as input
  vscG_i2dqRef : Outport
  wires:
  kidc/1 -> Discrete-Time Integrator1/1
  Grid Current Reference Calculation/1(vscG_i2dqRef) -> Scope1/1, vscG_i2dqRef/1
  vscG_egdq/1 -> Grid Current Reference Calculation/3(vscG_egdqPos)
  Constant1/1 -> Grid Current Reference Calculation/4(SNG_IMAXG)
  Logical Operator/1 -> Discrete-Time Integrator1/2
  [initDCControllerGrid_C1] -> Logical Operator/1
  [initDCControllerGrid_C1] -> Product1/1
  Product1/1 -> Grid Current Reference Calculation/2(vscG_pgRef)
  Constant3/1 -> Switch1/2
  [vscG_PgRefAUX_C1] -> Switch1/3
  Sum5/1 -> kpdc1/1
  Product3/1 -> Sum5/2
  Product2/1 -> Sum5/1
  vscG_vdc/1 -> Product3/1, Product3/2
  kpdc/1 -> Sum2/2
  Discrete-Time Integrator1/1 -> Scope3/1, Sum2/1
  Sum7/1 -> kidc/1
  Sum2/1 -> Sum4/2, Scope2/1, Switch1/1
  Sum4/1 -> kawcdc/1
  kawcdc/1 -> Sum7/1
  Grid Current Reference Calculation/2(Pg) -> Sum4/1
  vscG_qgRef/1 -> Grid Current Reference Calculation/1(vscG_qgRef)
  Switch1/1 -> Product1/2
  kpdc1/1 -> Sum7/2, kpdc/1
  Rate Limiter/1 -> Scope4/1, Product2/2, Product2/1
  [vscG_VdcRef_C1] -> Product4/1
  [initDCControllerGrid_C1] -> Product4/2
  Product4/1 -> Saturation1/1
  Saturation1/1 -> Rate Limiter/1

== system B2B_2x15kW_LCO_paralelo_y_serie/VSC1 Controller2/Grid Side Measurements ==
  vscG_i1abc : Inport
  vscG_i2abc : Inport  Port=2
  vscG_egabc : Inport  Port=3
  vscG_vdc_ : Inport  Port=4
  D-LCO FLL : Subsystem
  abc to dq eg : Subsystem
  abc to dq i1 : Subsystem
  abc to dq i2 : Subsystem
  udc measurement : Subsystem
  vscG_i1dq : Outport
  vscG_i2dq : Outport  Port=2
  vscG_egdqPos : Outport  Port=3  SampleTime=TS_C
  vscG_thetaPLL : Outport  Port=4  SampleTime=TS_C
  vscG_vdc : Outport  Port=5
  vscG_egdq : Outport  Port=6
  vscG_omegaPLL : Outport  Port=7  SampleTime=TS_C
  wires:
  vscG_i1abc/1 -> abc to dq i1/1(vscG_i1abc)
  vscG_egabc/1 -> abc to dq eg/1(vscG_egabc), D-LCO FLL/1(vscG_egabc)
  vscG_i2abc/1 -> abc to dq i2/1(vscG_i2abc)
  D-LCO FLL/2(vscG_egdqPos) -> vscG_egdqPos/1
  vscG_vdc_/1 -> udc measurement/1(vscG_vdc_)
  udc measurement/1(vscG_vdc) -> vscG_vdc/1
  abc to dq eg/1(vscG_egdq) -> vscG_egdq/1
  D-LCO FLL/3(vscG_omegaPLL) -> vscG_omegaPLL/1
  abc to dq i2/1(vscG_i2dq) -> vscG_i2dq/1
  abc to dq i1/1(vscG_i1dq) -> vscG_i1dq/1
  D-LCO FLL/1(vscG_thetaPLL) -> vscG_thetaPLL/1, abc to dq eg/2(vscG_theta), abc to dq i2/2(vscG_theta), abc to dq i1/2(vscG_theta)

== system B2B_2x15kW_LCO_paralelo_y_serie/VSC1 Controller2/Normalizacion ==
  vscG_ugabcActD : Inport
  vscG_vdc : Inport  Port=2
  Demux : Demux  Outputs=3
  Fcn : Fcn  Expr=2*u[1]/(u[2]+eps)
  Fcn1 : Fcn  Expr=2*u[1]/(u[2]+eps)
  Fcn2 : Fcn  Expr=2*u[1]/(u[2]+eps)
  Filter vdc : Subsystem
  Gain1 : Gain  Gain=1/2  SaturateOnIntegerOverflow=on  OutDataTypeStr=Inherit: Same as input  ParamDataTypeStr=Inherit: Same as input
  Manual Switch : ManualSwitch  CurrentSetting=0
  MinMax : MinMax  Function=max  Inputs=3  InputSameDT=on  SaturateOnIntegerOverflow=on
  MinMax2 : MinMax  Inputs=3  InputSameDT=on  SaturateOnIntegerOverflow=on
  Mux1 : Mux  Inputs=2
  Mux2 : Mux  Inputs=2
  Mux3 : Mux  Inputs=2
  Mux4 : Mux  Inputs=3
  Mux5 : Mux  Inputs=3
  Sum2 : Sum  InputSameDT=on  SaturateOnIntegerOverflow=on  OutDataTypeStr=Inherit: Same as first input
  Sum3 : Sum  Inputs=+-  InputSameDT=on  SaturateOnIntegerOverflow=on  OutDataTypeStr=Inherit: Same as first input
  Sum4 : Sum  Inputs=+-  InputSameDT=on  SaturateOnIntegerOverflow=on  OutDataTypeStr=Inherit: Same as first input
  Sum5 : Sum  Inputs=+-  InputSameDT=on  SaturateOnIntegerOverflow=on  OutDataTypeStr=Inherit: Same as first input
  vscG_dabc : Outport
  wires:
  vscG_vdc/1 -> Filter vdc/1(vscG_vdc)
  Sum3/1 -> Mux4/1  "vscG_pwmA"
  Sum4/1 -> Mux4/2  "vscG_pwmB"
  Sum5/1 -> Mux4/3  "vscG_pwmC"
  MinMax/1 -> Sum2/1
  MinMax2/1 -> Sum2/2
  Sum2/1 -> Gain1/1
  Fcn/1 -> Mux5/1, Sum3/1, MinMax2/1, MinMax/1
  Fcn2/1 -> MinMax/3, MinMax2/3, Sum5/1, Mux5/3
  Fcn1/1 -> Mux5/2, MinMax/2, MinMax2/2, Sum4/1
  Mux1/1 -> Fcn/1
  Mux2/1 -> Fcn1/1
  Mux3/1 -> Fcn2/1
  Demux/2 -> Mux2/1
  Demux/3 -> Mux3/1
  Demux/1 -> Mux1/1
  Gain1/1 -> Sum3/2, Sum4/2, Sum5/2
  Filter vdc/1(Out) -> Mux3/2, Mux1/2, Mux2/2
  vscG_ugabcActD/1 -> Demux/1
  Mux4/1 -> Manual Switch/2
  Mux5/1 -> Manual Switch/1
  Manual Switch/1 -> vscG_dabc/1

== system B2B_2x15kW_LCO_paralelo_y_serie/VSC1 Controller2/State Machine ==
  Constant2 : Constant  Value=dataStateMachine  SampleTime=TS_C
  Constant6 : Constant  SampleTime=TS_C
  Constant8 : Constant  Value=0  SampleTime=TS_C
  Demux : Demux  Outputs=8
  Logic detection : Subsystem
  Mux : Mux  Inputs=6
  Scope2 : Scope
      settings: ActiveDisplayYMinimum=0  ActiveDisplayYMaximum=2100  DataLoggingVariableName=ScopeData12
  Scope3 : Scope
      settings: ActiveDisplayYMinimum=1.9  ActiveDisplayYMaximum=2.1  DataLoggingVariableName=ScopeData14
  State Machine : MATLAB Function  TreatAsAtomicUnit=on
  Unit Delay5 : UnitDelay  InitialCondition=zeros(1,Ncount)  SampleTime=TS_C
  Unit Delay7 : UnitDelay  InitialCondition=1  SampleTime=TS_C
  tag scope: CONNECT_GRID_CONTACT_C1=global, CONNECT_PRELOAD_CONTACT_C1=global, PWMOnGrid_C1=global, initCurrentControllerG_C1=global, initDCControllerGrid_C1=global, initPLLGrid_C1=global, initReactiveVoltageController_C1=global, selReactiveVoltageController_C1=global
  wires:
  State Machine/3(nowCounters) -> Unit Delay5/1, Scope2/1
  Mux/1 -> State Machine/2(inputs)
  Constant2/1 -> State Machine/1(data)
  Unit Delay5/1 -> State Machine/4(prevCounters)
  State Machine/2(nowState) -> Unit Delay7/1, Scope3/1
  Unit Delay7/1 -> State Machine/3(prevState)
  [MEAS_vscG_vdc_C1] -> Logic detection/1(vscG_vdc)
  State Machine/1(outputs) -> Demux/1
  [MEAS_vscG_egabc_C1] -> Logic detection/2(vscG_egabc)
  Demux/1 -> [PWMOnGrid_C1]
  Demux/2 -> [CONNECT_GRID_CONTACT_C1]
  Demux/3 -> [CONNECT_PRELOAD_CONTACT_C1]
  Demux/8 -> [initDCControllerGrid_C1]
  Demux/7 -> [initCurrentControllerG_C1]
  Demux/6 -> [initReactiveVoltageController_C1]
  Demux/5 -> [initPLLGrid_C1]
  Demux/4 -> [selReactiveVoltageController_C1]
  Constant6/1 -> Mux/1  "PRECHARGE"
  [INPUT_CONNECT_INT_C1] -> Mux/2  "CONNECT"
  Constant8/1 -> Mux/3
  Logic detection/1(VDC_READY) -> Mux/4
  Logic detection/2(VDC_STEATS) -> Mux/5
  Logic detection/3(FLAG_SAG) -> Mux/6

== system B2B_2x15kW_LCO_paralelo_y_serie/VSC1 Controller2/dq to abc ==
  vscG_ugdqRef : Inport
  vscG_egdqPos : Inport  Port=2
  vscG_theta : Inport  Port=3
  Constant : Constant  Value=[WN_G L12 I_MAX_G]  SampleTime=TS_C
  Constant1 : Constant  Value=WN_G  SampleTime=TS_C
  Mux : Mux  Inputs=2
  Scope3 : Scope
      settings: SampleTime=TS_C  TimeSpan=5  ActiveDisplayYMinimum=24681.8  ActiveDisplayYMaximum=27279.8  DataLoggingDecimation=5  DataLoggingVariableName=Variables_i2dq7  DataLoggingSaveFormat=Array
  Sum : Sum  Inputs=|++
  dq to abc : Subsystem  AncestorBlock=Transformations_blocks/dq2abc
  th advance : Gain  Gain=TS_C*5/2
  udq Limitation : MATLAB Function  TreatAsAtomicUnit=on
  vscG_ugabcSat : Outport
  vscG_ugdqSat : Outport  Port=2
  wires:
  dq to abc/1(vscG_ugabcSat) -> vscG_ugabcSat/1
  Sum/1 -> dq to abc/2(vsc_thetaAdvanced)
  vscG_theta/1 -> Sum/1
  th advance/1 -> Sum/2
  Constant1/1 -> th advance/1
  Constant/1 -> udq Limitation/3(WNG_L12_IMAXG)
  vscG_egdqPos/1 -> udq Limitation/2(vscG_egdqPos)
  udq Limitation/1(vscG_ugdqSat) -> Mux/2, vscG_ugdqSat/1, dq to abc/1(vscG_ugdqSat)
  vscG_ugdqRef/1 -> Mux/1, udq Limitation/1(vscG_ugdqRef)
  Mux/1 -> Scope3/1

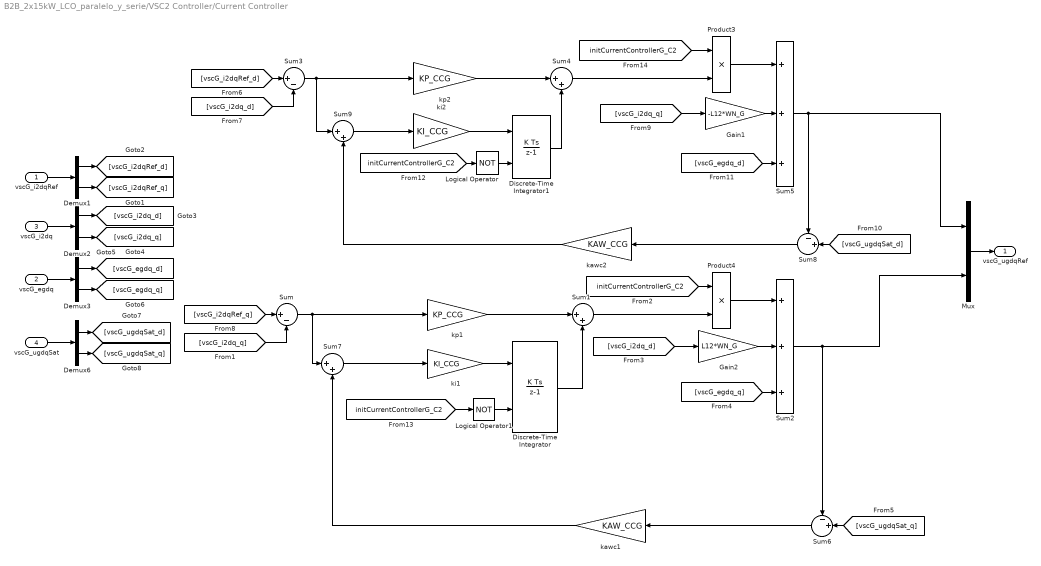
== system B2B_2x15kW_LCO_paralelo_y_serie/VSC2 Controller/Current Controller ==
  vscG_i2dqRef : Inport
  vscG_egdq : Inport  Port=2
  vscG_i2dq : Inport  Port=3
  vscG_ugdqSat : Inport  Port=4
  Demux{1..3,6} (4 alike) : Demux  Outputs=2
  Discrete-Time Integrator : DiscreteIntegrator  ExternalReset=level  SampleTime=-1  UpperSaturationLimit=sqrt(2/3)*750  LowerSaturationLimit=-sqrt(2/3)*750  ICPrevOutput=DiscIntNeverNeededParam  ICPrevScaledInput=DiscIntNeverNeededParam
  Discrete-Time Integrator1 : DiscreteIntegrator  ExternalReset=level  SampleTime=-1  UpperSaturationLimit=sqrt(2/3)*750  LowerSaturationLimit=-sqrt(2/3)*750  ICPrevOutput=DiscIntNeverNeededParam  ICPrevScaledInput=DiscIntNeverNeededParam
  Gain1 : Gain  Gain=-L12*WN_G  SaturateOnIntegerOverflow=on  OutDataTypeStr=Inherit: Same as input  ParamDataTypeStr=Inherit: Same as input
  Gain2 : Gain  Gain=L12*WN_G  SaturateOnIntegerOverflow=on  OutDataTypeStr=Inherit: Same as input  ParamDataTypeStr=Inherit: Same as input
  Logical Operator : Logic  Operator=NOT  AllPortsSameDT=off  OutDataTypeStr=boolean
  Logical Operator1 : Logic  Operator=NOT  AllPortsSameDT=off  OutDataTypeStr=boolean
  Mux : Mux  Inputs=2
  Product3 : Product  InputSameDT=on  SaturateOnIntegerOverflow=on  OutDataTypeStr=Inherit: Same as first input
  Product4 : Product  InputSameDT=on  SaturateOnIntegerOverflow=on  OutDataTypeStr=Inherit: Same as first input
  Sum : Sum  Inputs=|+-  InputSameDT=on  SaturateOnIntegerOverflow=on  OutDataTypeStr=Inherit: Same as first input
  Sum{1,4,7,9} (4 alike) : Sum  Inputs=|++  InputSameDT=on  SaturateOnIntegerOverflow=on  OutDataTypeStr=Inherit: Same as first input
  Sum2 : Sum  Inputs=+++  InputSameDT=on  SaturateOnIntegerOverflow=on  OutDataTypeStr=Inherit: Same as first input
  Sum3 : Sum  Inputs=|+-  InputSameDT=on  SaturateOnIntegerOverflow=on  OutDataTypeStr=Inherit: Same as first input
  Sum5 : Sum  Inputs=+++  InputSameDT=on  SaturateOnIntegerOverflow=on  OutDataTypeStr=Inherit: Same as first input
  Sum6 : Sum  Inputs=-+|  InputSameDT=on  SaturateOnIntegerOverflow=on  OutDataTypeStr=Inherit: Same as first input
  Sum8 : Sum  Inputs=-+|  InputSameDT=on  SaturateOnIntegerOverflow=on  OutDataTypeStr=Inherit: Same as first input
  kawc1 : Gain  Gain=KAW_CCG  SaturateOnIntegerOverflow=on  OutDataTypeStr=Inherit: Same as input  ParamDataTypeStr=Inherit: Same as input
  kawc2 : Gain  Gain=KAW_CCG  SaturateOnIntegerOverflow=on  OutDataTypeStr=Inherit: Same as input  ParamDataTypeStr=Inherit: Same as input
  ki1 : Gain  Gain=KI_CCG  SaturateOnIntegerOverflow=on  OutDataTypeStr=Inherit: Same as input  ParamDataTypeStr=Inherit: Same as input
  ki2 : Gain  Gain=KI_CCG  SaturateOnIntegerOverflow=on  OutDataTypeStr=Inherit: Same as input  ParamDataTypeStr=Inherit: Same as input
  kp1 : Gain  Gain=KP_CCG  SaturateOnIntegerOverflow=on  OutDataTypeStr=Inherit: Same as input  ParamDataTypeStr=Inherit: Same as input
  kp2 : Gain  Gain=KP_CCG  SaturateOnIntegerOverflow=on  OutDataTypeStr=Inherit: Same as input  ParamDataTypeStr=Inherit: Same as input
  vscG_ugdqRef : Outport
  wires:
  Mux/1 -> vscG_ugdqRef/1
  vscG_i2dq/1 -> Demux2/1
  vscG_egdq/1 -> Demux3/1
  Demux1/1 -> [vscG_i2dqRef_d]
  Demux1/2 -> [vscG_i2dqRef_q]
  Demux2/1 -> [vscG_i2dq_d]
  Demux3/2 -> [vscG_egdq_q]
  Demux3/1 -> [vscG_egdq_d]
  Demux2/2 -> [vscG_i2dq_q]
  vscG_i2dqRef/1 -> Demux1/1
  [vscG_i2dqRef_q] -> Sum/1
  ki1/1 -> Discrete-Time Integrator/1
  [vscG_egdq_q] -> Sum2/3
  Gain2/1 -> Sum2/2
  Sum/1 -> Sum7/1, kp1/1
  [vscG_i2dqRef_d] -> Sum3/1
  ki2/1 -> Discrete-Time Integrator1/1
  Gain1/1 -> Sum5/2
  [vscG_egdq_d] -> Sum5/3
  [vscG_i2dq_q] -> Gain1/1
  Sum3/1 -> Sum9/1, kp2/1
  Logical Operator/1 -> Discrete-Time Integrator1/2
  [initCurrentControllerG_C2] -> Logical Operator/1
  [initCurrentControllerG_C2] -> Logical Operator1/1
  Logical Operator1/1 -> Discrete-Time Integrator/2
  Sum4/1 -> Product3/2
  Product3/1 -> Sum5/1
  [initCurrentControllerG_C2] -> Product3/1
  Product4/1 -> Sum2/1
  Sum1/1 -> Product4/2
  [initCurrentControllerG_C2] -> Product4/1
  [vscG_i2dq_d] -> Sum3/2
  [vscG_i2dq_q] -> Sum/2
  [vscG_i2dq_d] -> Gain2/1
  kp1/1 -> Sum1/1
  Discrete-Time Integrator/1 -> Sum1/2
  Discrete-Time Integrator1/1 -> Sum4/2
  kp2/1 -> Sum4/1
  Sum5/1 -> Sum8/1, Mux/1
  [vscG_ugdqSat_d] -> Sum8/2
  Sum8/1 -> kawc2/1
  Sum9/1 -> ki2/1
  kawc2/1 -> Sum9/2
  Sum2/1 -> Sum6/1, Mux/2
  [vscG_ugdqSat_q] -> Sum6/2
  Sum6/1 -> kawc1/1
  kawc1/1 -> Sum7/2
  Sum7/1 -> ki1/1
  vscG_ugdqSat/1 -> Demux6/1
  Demux6/1 -> [vscG_ugdqSat_d]
  Demux6/2 -> [vscG_ugdqSat_q]

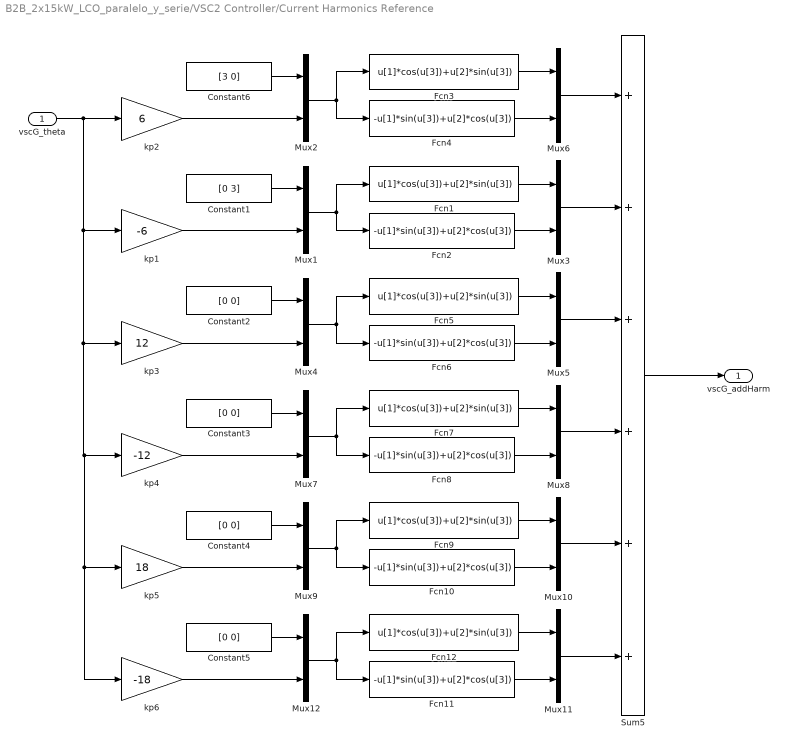
== system B2B_2x15kW_LCO_paralelo_y_serie/VSC2 Controller/Current Harmonics Reference ==
  vscG_theta : Inport  SampleTime=TS_C
  Constant1 : Constant  Value=[0 3]  SampleTime=TS_C
  Constant{2..5} (4 alike) : Constant  Value=[0 0]  SampleTime=TS_C
  Constant6 : Constant  Value=[3 0]  SampleTime=TS_C
  Fcn{1,3,5,7,9,12} (6 alike) : Fcn  Expr=u[1]*cos(u[3])+u[2]*sin(u[3])
  Fcn{2,4,6,8,10..11} (6 alike) : Fcn  Expr=-u[1]*sin(u[3])+u[2]*cos(u[3])
  Mux{1..12} (12 alike) : Mux  Inputs=2
  Sum5 : Sum  Inputs=++++++  InputSameDT=on  SaturateOnIntegerOverflow=on  OutDataTypeStr=Inherit: Same as first input
  kp1 : Gain  Gain=-6  SaturateOnIntegerOverflow=on  OutDataTypeStr=Inherit: Same as input  ParamDataTypeStr=Inherit: Same as input
  kp2 : Gain  Gain=6  SaturateOnIntegerOverflow=on  OutDataTypeStr=Inherit: Same as input  ParamDataTypeStr=Inherit: Same as input
  kp3 : Gain  Gain=12  SaturateOnIntegerOverflow=on  OutDataTypeStr=Inherit: Same as input  ParamDataTypeStr=Inherit: Same as input
  kp4 : Gain  Gain=-12  SaturateOnIntegerOverflow=on  OutDataTypeStr=Inherit: Same as input  ParamDataTypeStr=Inherit: Same as input
  kp5 : Gain  Gain=18  SaturateOnIntegerOverflow=on  OutDataTypeStr=Inherit: Same as input  ParamDataTypeStr=Inherit: Same as input
  kp6 : Gain  Gain=-18  SaturateOnIntegerOverflow=on  OutDataTypeStr=Inherit: Same as input  ParamDataTypeStr=Inherit: Same as input
  vscG_addHarm : Outport
  wires:
  Mux2/1 -> Fcn4/1, Fcn3/1
  Fcn3/1 -> Mux6/1
  Fcn4/1 -> Mux6/2
  Constant6/1 -> Mux2/1
  kp2/1 -> Mux2/2
  Mux6/1 -> Sum5/1
  Sum5/1 -> vscG_addHarm/1
  Mux1/1 -> Fcn1/1, Fcn2/1
  Fcn1/1 -> Mux3/1
  Fcn2/1 -> Mux3/2
  Constant1/1 -> Mux1/1
  vscG_theta/1 -> kp6/1, kp5/1, kp4/1, kp3/1, kp1/1, kp2/1
  Mux3/1 -> Sum5/2
  kp1/1 -> Mux1/2
  Mux4/1 -> Fcn6/1, Fcn5/1
  Fcn5/1 -> Mux5/1
  Fcn6/1 -> Mux5/2
  Constant2/1 -> Mux4/1
  Mux5/1 -> Sum5/3
  kp3/1 -> Mux4/2
  Mux7/1 -> Fcn7/1, Fcn8/1
  Fcn7/1 -> Mux8/1
  Fcn8/1 -> Mux8/2
  Constant3/1 -> Mux7/1
  kp4/1 -> Mux7/2
  Mux8/1 -> Sum5/4
  Mux9/1 -> Fcn10/1, Fcn9/1
  Fcn9/1 -> Mux10/1
  Fcn10/1 -> Mux10/2
  Constant4/1 -> Mux9/1
  kp5/1 -> Mux9/2
  Mux10/1 -> Sum5/5
  Mux12/1 -> Fcn12/1, Fcn11/1
  Fcn12/1 -> Mux11/1
  Fcn11/1 -> Mux11/2
  Constant5/1 -> Mux12/1
  kp6/1 -> Mux12/2
  Mux11/1 -> Sum5/6
